simulink subsystem "wheelSlip"  (R2022b)
settings: Solver=VariableStepAuto  StartTime=0.0  StopTime=10.0  RelTol=1e-3
libraries: wheels x3
settings Model: Creator=serga  LastModifiedBy=serga

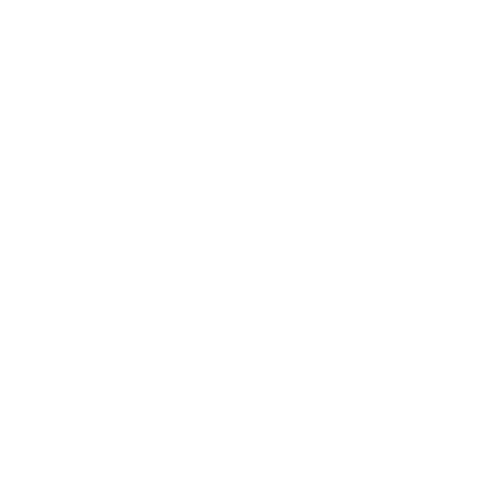
[thumbnail: Simulink's stored preview of the top-level diagram]
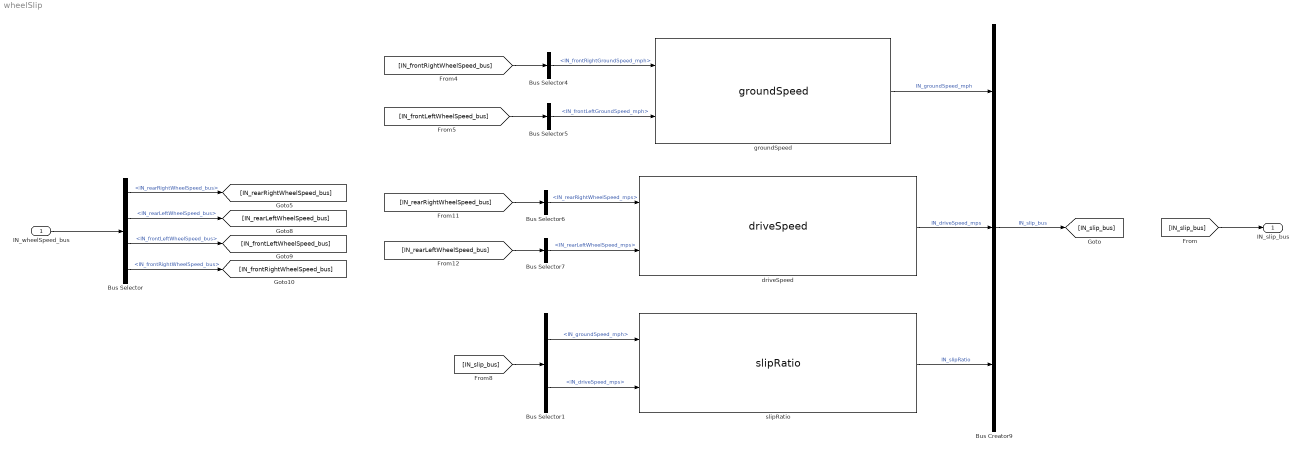
== system wheelSlip ==
  IN_wheelSpeed_bus : Inport
  Bus Creator9 : BusCreator  Inputs=3
  Bus Selector : BusSelector  OutputSignals=IN_rearRightWheelSpeed_bus,IN_rearLeftWheelSpeed_bus,IN_frontLeftWheelSpeed_bus,IN_frontRightWheelSpeed_bus
  Bus Selector1 : BusSelector  OutputSignals=IN_groundSpeed_mph,IN_driveSpeed_mps
  Bus Selector4 : BusSelector  OutputSignals=IN_frontRightGroundSpeed_mph
  Bus Selector5 : BusSelector  OutputSignals=IN_frontLeftGroundSpeed_mph
  Bus Selector6 : BusSelector  OutputSignals=IN_rearRightWheelSpeed_mps
  Bus Selector7 : BusSelector  OutputSignals=IN_rearLeftWheelSpeed_mps
  driveSpeed : wheels/driveSpeed  SystemSampleTime=-1  VariantActivationTime=update diagram  Latency=0  AutoFrameSizeCalculation=off
  groundSpeed : wheels/groundSpeed  SystemSampleTime=-1  VariantActivationTime=update diagram  Latency=0  AutoFrameSizeCalculation=off
  slipRatio : wheels/slipRatio  SystemSampleTime=-1  VariantActivationTime=update diagram  Latency=0  AutoFrameSizeCalculation=off
  IN_slip_bus : Outport
  wires:
  Bus Selector1/1 -> slipRatio/1  "<IN_groundSpeed_mph>"
  slipRatio/1 -> Bus Creator9/3  "IN_slipRatio"
  Bus Selector1/2 -> slipRatio/2  "<IN_driveSpeed_mps>"
  Bus Selector/2 -> [IN_rearLeftWheelSpeed_bus]  "<IN_rearLeftWheelSpeed_bus>"
  Bus Selector6/1 -> driveSpeed/1  "<IN_rearRightWheelSpeed_mps>"
  [IN_slip_bus] -> Bus Selector1/1
  Bus Selector7/1 -> driveSpeed/2  "<IN_rearLeftWheelSpeed_mps>"
  Bus Selector/1 -> [IN_rearRightWheelSpeed_bus]  "<IN_rearRightWheelSpeed_bus>"
  groundSpeed/1 -> Bus Creator9/1  "IN_groundSpeed_mph"
  Bus Creator9/1 -> [IN_slip_bus]  "IN_slip_bus"
  Bus Selector/3 -> [IN_frontLeftWheelSpeed_bus]  "<IN_frontLeftWheelSpeed_bus>"
  Bus Selector/4 -> [IN_frontRightWheelSpeed_bus]  "<IN_frontRightWheelSpeed_bus>"
  [IN_frontLeftWheelSpeed_bus] -> Bus Selector5/1
  IN_wheelSpeed_bus/1 -> Bus Selector/1
  [IN_frontRightWheelSpeed_bus] -> Bus Selector4/1
  driveSpeed/1 -> Bus Creator9/2  "IN_driveSpeed_mps"
  Bus Selector4/1 -> groundSpeed/1  "<IN_frontRightGroundSpeed_mph>"
  [IN_rearLeftWheelSpeed_bus] -> Bus Selector7/1
  [IN_rearRightWheelSpeed_bus] -> Bus Selector6/1
  Bus Selector5/1 -> groundSpeed/2  "<IN_frontLeftGroundSpeed_mph>"
  [IN_slip_bus] -> IN_slip_bus/1
